simulink model "pressure_controller_harness"  (R2025b)
settings: Solver=VariableStepAuto  StartTime=0.0  StopTime=10.0  RelTol=1e-3
InitFcn:
  | controller_mode = controller_modes.PRESSURE
settings Model: Creator=karadeli  LastModifiedBy=Kaan Kalkandelen

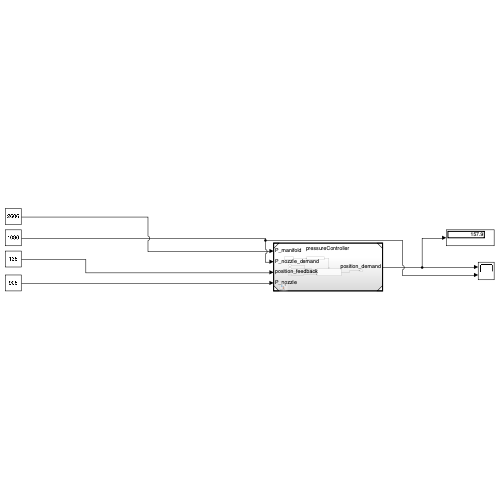
[thumbnail: Simulink's stored preview of the top-level diagram]
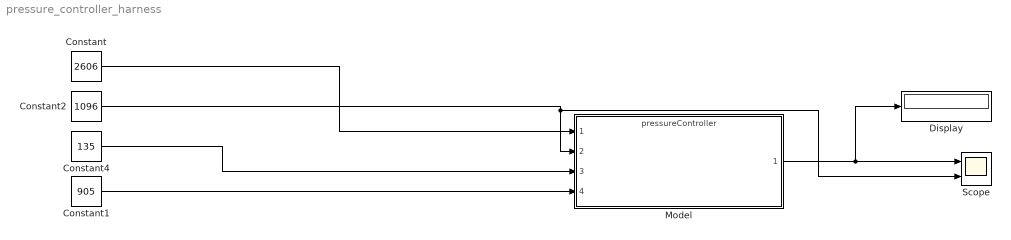
== system pressure_controller_harness ==
  Constant : Constant  Value=2606  OutDataTypeStr=single
  Constant1 : Constant  Value=905  OutDataTypeStr=single
  Constant2 : Constant  Value=1096  OutDataTypeStr=single
  Constant4 : Constant  Value=135  OutDataTypeStr=single
  Display : Display
  Model : ModelReference  ModelNameDialog=pressureController.slx  SimulationMode=Normal  ModelReferenceVersion=1.20
  Scope : Scope  NumInputPorts=2
      settings: ActiveDisplayYMinimum=-134.99999999999997  ActiveDisplayYMaximum=1215
  wires:
  Constant/1 -> Model/1
  Model/1 -> Scope/1, Display/1
  Constant2/1 -> Model/2, Scope/2
  Constant4/1 -> Model/3
  Constant1/1 -> Model/4
